simulink model "ObjectPP"  (R2023b)
settings: Solver=VariableStepAuto  StartTime=0.0  StopTime=inf  RelTol=1e-3
libraries: simulink x7, ros2lib x2, rllib x1
settings Model: Creator=cgpda  LastModifiedBy=paul

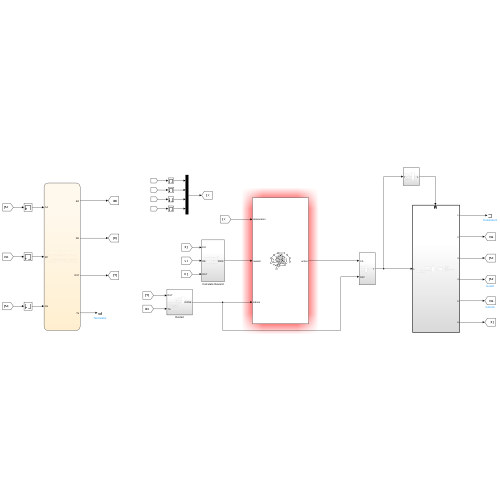
[thumbnail: Simulink's stored preview of the top-level diagram]
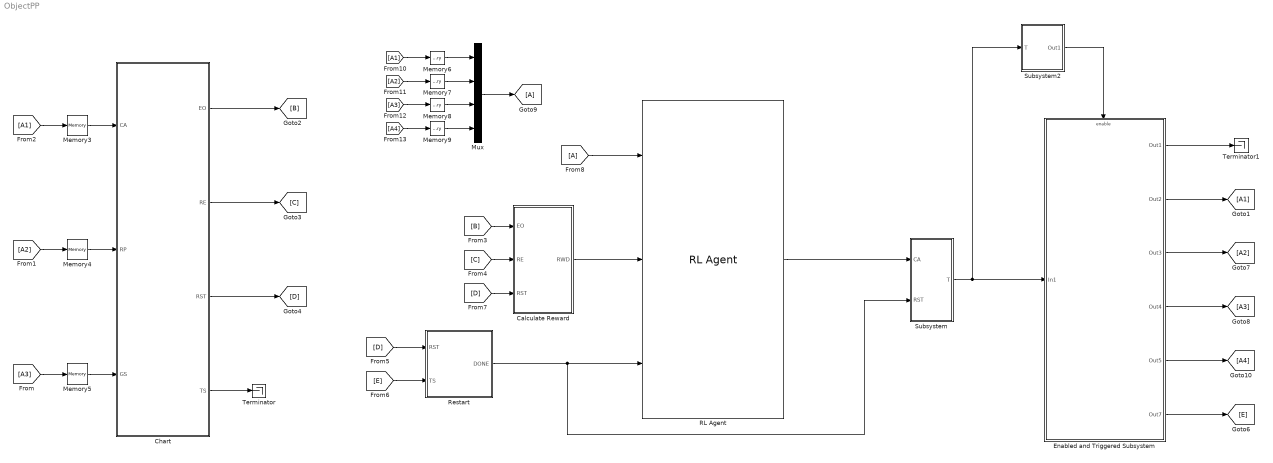
== system ObjectPP ==
  Calculate Reward : Subsystem
  Chart : Stateflow chart  TreatAsAtomicUnit=on
  Enabled and Triggered Subsystem : Subsystem  TreatAsAtomicUnit=on
  From8 : From
  Goto9 : Goto
  Memory{3..8} (6 alike) : Memory  InitialCondition=1
  Memory9 : Memory
  Mux : Mux
  RL Agent : rllib/RL Agent  Agent=agent1  ExternalActionAsInput=off  ProvideLastAction=off  ProvideCumRwd=off  TreatAsDirectFeedthrough=on  UseStrictObservationDataTypes=off
  Restart : Subsystem
  Subsystem : Subsystem
  Subsystem2 : Subsystem
  Terminator : Terminator
  Terminator1 : Terminator
  wires:
  [A3] -> Memory5/1
  [A2] -> Memory4/1
  [A1] -> Memory3/1
  From8/1 -> RL Agent/1
  [C] -> Calculate Reward/2(RE)
  [D] -> Restart/1(RST)
  [B] -> Calculate Reward/1(EO)
  [E] -> Restart/2(TS)
  Calculate Reward/1(RWD) -> RL Agent/2
  [D] -> Calculate Reward/3(RST)
  [A4] -> Memory9/1
  [A3] -> Memory8/1
  [A2] -> Memory7/1
  [A1] -> Memory6/1
  Mux/1 -> Goto9/1
  Memory3/1 -> Chart/1(CA)
  Memory4/1 -> Chart/2(RP)
  Memory5/1 -> Chart/3(GS)
  Memory6/1 -> Mux/1
  Memory7/1 -> Mux/2
  Memory8/1 -> Mux/3
  Memory9/1 -> Mux/4
  Chart/3(RST) -> [D]
  Chart/2(RE) -> [C]
  Chart/1(EO) -> [B]
  Chart/4(TS) -> Terminator/1
  Enabled and Triggered Subsystem/4(Out4) -> [A3]
  Enabled and Triggered Subsystem/3(Out3) -> [A2]
  Subsystem/1(T) -> Enabled and Triggered Subsystem/1(In1), Subsystem2/1(T)
  Enabled and Triggered Subsystem/2(Out2) -> [A1]
  RL Agent/1 -> Subsystem/1(CA)
  Restart/1(DONE) -> Subsystem/2(RST), RL Agent/3
  Subsystem2/1(Out1) -> Enabled and Triggered Subsystem/Enable
  Enabled and Triggered Subsystem/6(Out7) -> [E]
  Enabled and Triggered Subsystem/5(Out5) -> [A4]
  Enabled and Triggered Subsystem/1(Out1) -> Terminator1/1

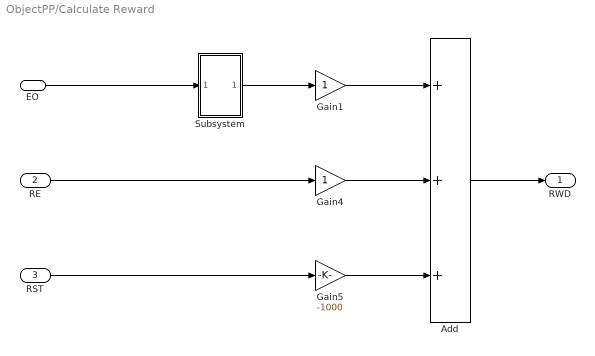
== system ObjectPP/Calculate Reward ==
  EO : Inport
  RE : Inport  Port=2
  RST : Inport  Port=3
  Add : Sum  Inputs=+++
  Gain1 : Gain
  Gain4 : Gain
  Gain5 : Gain  Gain=-1000
  Subsystem : Subsystem
  RWD : Outport
  wires:
  Add/1 -> RWD/1
  RST/1 -> Gain5/1
  Gain5/1 -> Add/3
  Gain1/1 -> Add/1
  EO/1 -> Subsystem/1(In1)
  Subsystem/1(Out1) -> Gain1/1
  Gain4/1 -> Add/2
  RE/1 -> Gain4/1

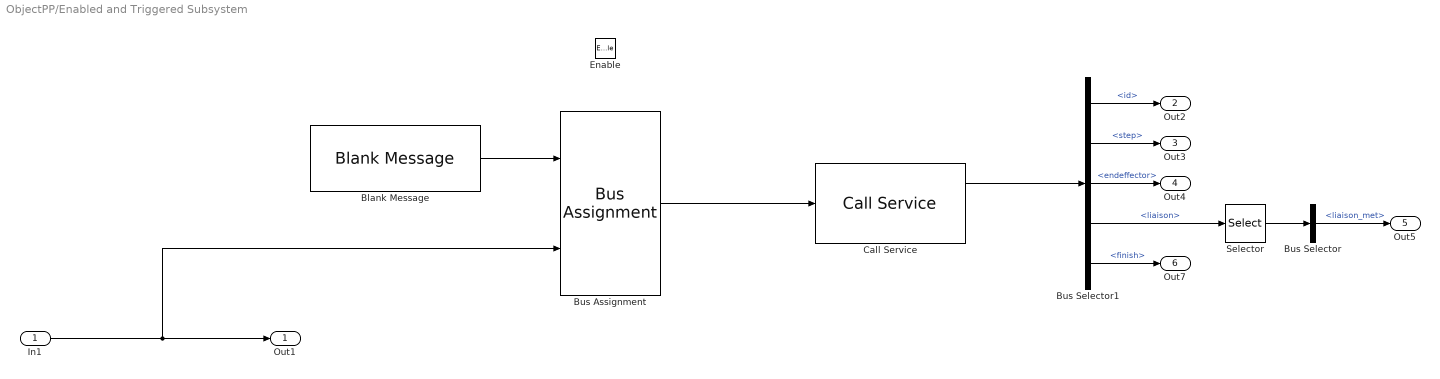
== system ObjectPP/Enabled and Triggered Subsystem ==
  In1 : Inport
  Enable : EnablePort
  Blank Message : ros2lib/Blank Message  messageClass=Service Request  entityType=r3m_data/SkillExecution  messageType=r3m_data/SkillExecutionRequest  SampleTime=-1
  Bus Assignment : BusAssignment  AssignedSignals=id
  Bus Selector : BusSelector  OutputSignals=liaison_met
  Bus Selector1 : BusSelector  OutputSignals=result.id,result.robstate.step,result.robstate.endeffector,result.liaison,result.finish
  Call Service : ros2lib/Call Service  topicSource=Select from ROS network  service=/r3m_SkillExecution  serviceType=r3m_data/SkillExecution  connectionTimeout=100  ShowErrorCodeOutput=on  legacyBusStruct=off  QOSHistory=Keep last  QOSDepth=100  QOSReliability=Reliable  QOSDurability=Volatile
  Selector : Selector  InputPortWidth=16  IndexOptions=Index vector (dialog)  Indices=[1]  OutputSizes=1
  Out1 : Outport
  Out2 : Outport  Port=2
  Out3 : Outport  Port=3
  Out4 : Outport  Port=4
  Out5 : Outport  Port=5
  Out7 : Outport  Port=6
  wires:
  Blank Message/1 -> Bus Assignment/1
  Bus Assignment/1 -> Call Service/1
  In1/1 -> Out1/1, Bus Assignment/2
  Selector/1 -> Bus Selector/1
  Bus Selector1/2 -> Out3/1  "<step>"
  Bus Selector1/5 -> Out7/1  "<finish>"
  Bus Selector1/3 -> Out4/1  "<endeffector>"
  Bus Selector1/4 -> Selector/1  "<liaison>"
  Bus Selector1/1 -> Out2/1  "<id>"
  Bus Selector/1 -> Out5/1  "<liaison_met>"
  Call Service/1 -> Bus Selector1/1

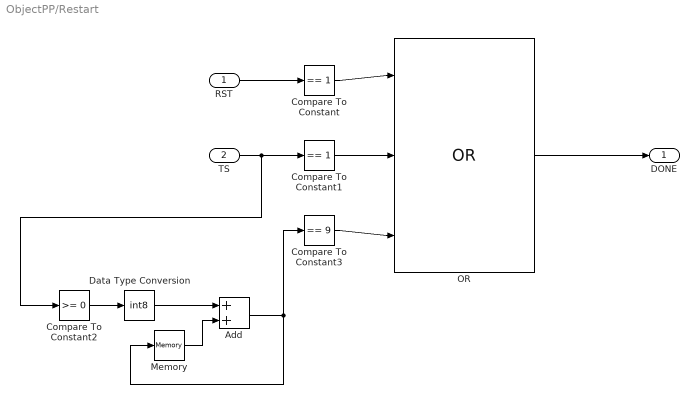
== system ObjectPP/Restart ==
  RST : Inport
  TS : Inport  Port=2
  Add : Sum
  Compare To Constant : simulink/Logic and Bit Operations/Compare To Constant  relop===  const=1  OutDataTypeStr=boolean
  Compare To Constant1 : simulink/Logic and Bit Operations/Compare To Constant  relop===  const=1  OutDataTypeStr=boolean
  Compare To Constant2 : simulink/Logic and Bit Operations/Compare To Constant  relop=>=  const=0  OutDataTypeStr=boolean
  Compare To Constant3 : simulink/Logic and Bit Operations/Compare To Constant  relop===  const=9  OutDataTypeStr=boolean
  Data Type Conversion : DataTypeConversion  OutDataTypeStr=int8  SaturateOnIntegerOverflow=off  RndMeth=Floor
  Memory : Memory
  OR : Logic  Operator=OR  Inputs=3  IconShape=distinctive  AllPortsSameDT=off  OutDataTypeStr=boolean
  DONE : Outport
  wires:
  Compare To Constant2/1 -> Data Type Conversion/1
  OR/1 -> DONE/1
  RST/1 -> Compare To Constant/1
  Add/1 -> Compare To Constant3/1, Memory/1
  Data Type Conversion/1 -> Add/1
  Compare To Constant/1 -> OR/1
  Compare To Constant3/1 -> OR/3
  Memory/1 -> Add/2
  TS/1 -> Compare To Constant1/1, Compare To Constant2/1
  Compare To Constant1/1 -> OR/2

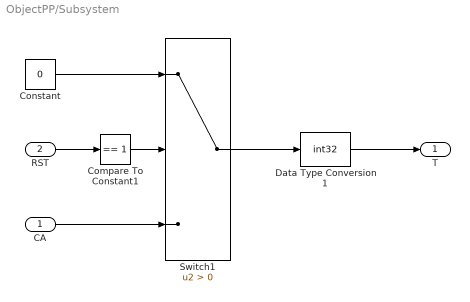
== system ObjectPP/Subsystem ==
  CA : Inport
  RST : Inport  Port=2
  Compare To Constant1 : simulink/Logic and Bit Operations/Compare To Constant  relop===  const=1  OutDataTypeStr=boolean
  Constant : Constant  Value=0  SampleTime=-1
  Data Type Conversion1 : DataTypeConversion  OutMin=[0]  OutMax=[7]  OutDataTypeStr=int32  SaturateOnIntegerOverflow=off  RndMeth=Floor
  Switch1 : Switch  Criteria=u2 > Threshold  SaturateOnIntegerOverflow=off  InputSameDT=off
  T : Outport
  wires:
  Data Type Conversion1/1 -> T/1
  Switch1/1 -> Data Type Conversion1/1
  RST/1 -> Compare To Constant1/1
  Compare To Constant1/1 -> Switch1/2
  CA/1 -> Switch1/3
  Constant/1 -> Switch1/1

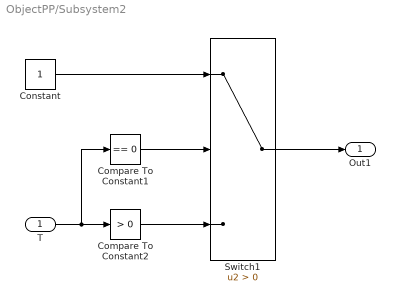
== system ObjectPP/Subsystem2 ==
  T : Inport
  Compare To Constant1 : simulink/Logic and Bit Operations/Compare To Constant  relop===  const=0  OutDataTypeStr=boolean
  Compare To Constant2 : simulink/Logic and Bit Operations/Compare To Constant  relop=>  const=0  OutDataTypeStr=boolean
  Constant : Constant  SampleTime=-1
  Switch1 : Switch  Criteria=u2 > Threshold  SaturateOnIntegerOverflow=off  InputSameDT=off
  Out1 : Outport
  wires:
  Constant/1 -> Switch1/1
  Compare To Constant1/1 -> Switch1/2
  T/1 -> Compare To Constant2/1, Compare To Constant1/1
  Switch1/1 -> Out1/1
  Compare To Constant2/1 -> Switch1/3

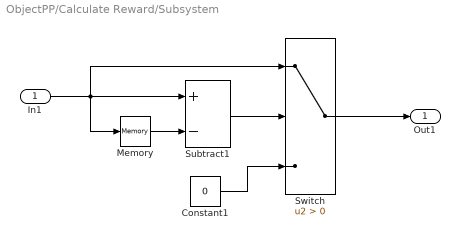
== system ObjectPP/Calculate Reward/Subsystem ==
  In1 : Inport
  Constant1 : Constant  Value=0
  Memory : Memory
  Subtract1 : Sum  Inputs=+-
  Switch : Switch  Criteria=u2 > Threshold  SaturateOnIntegerOverflow=off  InputSameDT=off
  Out1 : Outport
  wires:
  Memory/1 -> Subtract1/2
  Constant1/1 -> Switch/3
  Subtract1/1 -> Switch/2
  In1/1 -> Memory/1, Switch/1, Subtract1/1
  Switch/1 -> Out1/1

== stateflow chart ObjectPP/Chart ==
  state ProductState [parallel]
    settings: executionOrder=1
    state PartDropped
      entry, during:
      RST=0; TS=0;
    state ProductInitialState
      entry, during:
      RST=0; TS=0;
    state SkillReq1Completed
      entry, during:
      RST=0; TS=0;
    state SkillReq2Completed
      entry, during:
      RST=0; TS=0;
    state SkillReq3Completed
      entry, during:
      RST=0; TS=0;
    state SkillReq4Completed
      entry, during:
      RST=0; TS=0;
    state SkillReq5Completed
      entry, during:
      RST=0; TS=0;
    state SkillReq6Completed
      entry, during:
      RST=0; TS=0;
    state SkillReq7Completed
      entry, during:
      RST=0; TS=0;
    state SkillReq8Completed
      entry, during:
      RST=0; TS=0;
    state SkillReq9Completed1
      entry, during:
      RST=0; TS=0;
    ProductState.SkillReq5Completed -> PartDropped [order 2] : [GS==1]
    ProductState.SkillReq4Completed -> PartDropped [order 2] : [GS==1]
    (default) -> ProductState.ProductInitialState
    ProductState.SkillReq5Completed -> ProductState.SkillReq6Completed [order 1] : [RP==5 && GS==0]
    ProductState.SkillReq7Completed -> ProductState.SkillReq8Completed : [RP==4 && GS==1]
    ProductState.SkillReq8Completed -> SkillReq9Completed1 : [RP==1 && GS==1]
    ProductState.SkillReq1Completed -> ProductState.SkillReq2Completed : [RP==3 && GS==1]
    ProductState.ProductInitialState -> ProductState.SkillReq1Completed : [RP==2 && GS==1]
    ProductState.SkillReq2Completed -> ProductState.SkillReq3Completed : [RP==3 && GS==0]
    ProductState.SkillReq4Completed -> ProductState.SkillReq5Completed [order 1] : [RP==4 && GS==0]
    ProductState.SkillReq3Completed -> ProductState.SkillReq4Completed : [RP==2 && GS==0]
    ProductState.SkillReq6Completed -> ProductState.SkillReq7Completed : [RP==5 && GS==1]
  state ProductRequirements2 [parallel]
    settings: executionOrder=2
    state RecipeError1
      entry, during:
      RE=-500;
    state RecipeError2
      entry, during:
      RE=-500;
    state RecipeError3
      entry, during:
      RE=-500;
    state RecipeError4
      entry, during:
      RE=-500;
    state RecipeError5
      entry, during:
      RE=-500;
    state RecipeError6
      entry, during:
      RE=-500;
    state RecipeError7
      entry, during:
      RE=-500;
    state RecipeError8
      entry, during:
      RE=-500;
    state RecipeError9
      entry, during:
      RE=-500;
    state ProductInitialState
      entry, during:
      RE=0; EO=0;
    state SkillReq1Completed
      entry, during:
      RE=0; EO=100;
    state SkillReq2Completed
      entry, during:
      RE=0; EO=200;
    state SkillReq3Completed
      entry, during:
      RE=0; EO=300;
    state SkillReq4Completed
      entry, during:
      RE=0; EO=400;
    state SkillReq5Completed
      entry, during:
      RE=0; EO=500;
    state SkillReq6Completed
      entry, during:
      RE=0; EO=600
    state SkillReq7Completed
      entry, during:
      RE=0; EO=700;
    state SkillReq8Completed
      entry, during:
      RE=0; EO=800;
    state SkillReq9Completed
      entry, during:
      RE=0; EO=900;
    ProductRequirements2.ProductInitialState -> RecipeError1 [order 2] : [CA~=2]
    ProductRequirements2.SkillReq1Completed -> RecipeError2 [order 2] : [CA~=3]
    ProductRequirements2.SkillReq2Completed -> RecipeError3 [order 2] : [CA~=6]
    ProductRequirements2.SkillReq3Completed -> RecipeError4 [order 2] : [CA~=2]
    ProductRequirements2.SkillReq4Completed -> RecipeError5 [order 2] : [CA~=4]
    ProductRequirements2.SkillReq6Completed -> RecipeError7 [order 2] : [CA~=7]
    ProductRequirements2.SkillReq7Completed -> RecipeError8 [order 2] : [CA~=4]
    ProductRequirements2.SkillReq8Completed -> RecipeError9 [order 2] : [CA~=1]
    ProductRequirements2.SkillReq5Completed -> RecipeError6 [order 2] : [CA~=5]
    RecipeError1 -> ProductRequirements2.SkillReq1Completed : [RP==2 && GS==1]
    RecipeError2 -> ProductRequirements2.SkillReq2Completed : [RP==3 && GS==1]
    RecipeError3 -> ProductRequirements2.SkillReq3Completed : [RP==3 && GS==0]
    RecipeError4 -> ProductRequirements2.SkillReq4Completed : [RP==2 && GS==0]
    RecipeError5 -> ProductRequirements2.SkillReq5Completed : [RP==4 && GS==0]
    RecipeError6 -> ProductRequirements2.SkillReq6Completed : [RP==5 && GS==0]
    RecipeError7 -> ProductRequirements2.SkillReq7Completed : [RP==5 && GS==1]
    RecipeError8 -> ProductRequirements2.SkillReq8Completed : [RP==4 && GS==1]
    RecipeError9 -> SkillReq9Completed : [RP==1 && GS==1]
    (default) -> ProductRequirements2.ProductInitialState
    ProductRequirements2.SkillReq5Completed -> ProductRequirements2.SkillReq6Completed [order 1] : [CA==5]
    ProductRequirements2.SkillReq7Completed -> ProductRequirements2.SkillReq8Completed [order 1] : [CA==4]
    ProductRequirements2.SkillReq8Completed -> SkillReq9Completed [order 1] : [CA==1]
    ProductRequirements2.SkillReq1Completed -> ProductRequirements2.SkillReq2Completed [order 1] : [CA==3]
    ProductRequirements2.ProductInitialState -> ProductRequirements2.SkillReq1Completed [order 1] : [CA==2]
    ProductRequirements2.SkillReq2Completed -> ProductRequirements2.SkillReq3Completed [order 1] : [CA==6]
    ProductRequirements2.SkillReq4Completed -> ProductRequirements2.SkillReq5Completed [order 1] : [CA==4]
    ProductRequirements2.SkillReq3Completed -> ProductRequirements2.SkillReq4Completed [order 1] : [CA==2]
    ProductRequirements2.SkillReq6Completed -> ProductRequirements2.SkillReq7Completed [order 1] : [CA==7]
  data: CA input; RP input; GS input; EO output; RE output; RST output; TS output
